simulink model "vertical_sim"  (R2019b)
settings: Solver=VariableStepAuto  StartTime=0.0  StopTime=10.0  RelTol=1e-3
values from neighbouring files (symbols this model uses):
  Fs = Fl-Fr    [main_rocketmodel.m]    (also in main_sim_rocket.m; rocket_model.m)
  g = 9.8    [main_rocketmodel.m]    (also in main_sim_rocket.m; rocket_model.m; sim_lin.m; test_bangbang.m)
  m = 549054    [main_rocketmodel.m]    (also in main_sim_rocket.m; rocket_model.m = 25.4; sim_lin.m; test_bangbang.m)
  phi = (1e-6)*square(t_signal,25)    [main_rocketmodel.m]    (also in main_sim_rocket.m = zeros(length(t_signal),1); nominal_trajectory.m = zeros(length(t_signal),1); rocket_model.m = out.phi; sim_lin.m)
  theta = 0    [main_rocketmodel.m]    (also in main_sim_rocket.m; rocket_model.m)
settings Model: Creator=bia  LastModifiedBy=bia
settings DataIOCC: ExternalInput=[t, Fe]  LoadExternalInput=on

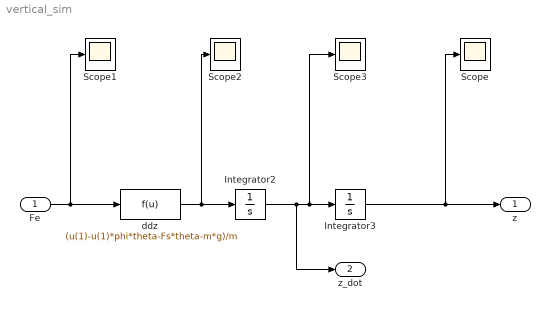
== system vertical_sim ==
  Fe : Inport
  Integrator2 : Integrator  ContinuousStateAttributes='z_dot'
  Integrator3 : Integrator  ContinuousStateAttributes='z'
  Scope{,1..3} (4 alike) : Scope
  ddz : Fcn  Expr=(u(1)-u(1)*phi*theta-Fs*theta-m*g)/m
  z : Outport
  "z_dot " : Outport  Port=2
  wires:
  Integrator3/1 -> Scope/1, z/1
  Integrator2/1 -> "z_dot "/1, Scope3/1, Integrator3/1
  ddz/1 -> Scope2/1, Integrator2/1
  Fe/1 -> Scope1/1, ddz/1
